simulink model "sim_tcyb_2024_att_ctrl"  (R2020a)
settings: Solver=ode4  StartTime=0.0  StopTime=30.0  FixedStep=0.01  RelTol=1e-3
values from neighbouring files (symbols this model uses):
  c1_diff_sigma_bar_w = diag([12; 12; 12])    [init_tcyb_2024_att_ctrl.m]
  c1_diff_ui = diag([25; 30; 20])    [init_tcyb_2024_att_ctrl.m]
  c2_diff_sigma_bar_w = diag([12; 12; 12])    [init_tcyb_2024_att_ctrl.m]
  c2_diff_ui = diag([50; 50; 10])    [init_tcyb_2024_att_ctrl.m]
  c3_diff_sigma_bar_w = diag([15; 15; 15])    [init_tcyb_2024_att_ctrl.m]
  c3_diff_ui = diag([15; 15; 10])    [init_tcyb_2024_att_ctrl.m]
  dw_aa_t = 0.2 * ones(3, 5) + ( 1.0 - 0.2 ) * rand(3, 5)    [init_tcyb_2024_att_ctrl.m]
  dw_ff_t = [ 0.4 * ones(1, 5) + ( 1.0 - 0.4 ) * rand(1, 5);                      0.4 * ones(1, 5) + ( 1.0 - 0.4 ) * rand(1, 5);                      0.2 * ones(1, 5) + ( 0.6 - 0.2 ) * rand(1, 5) ]    [init_tcyb_2024_att_ctrl.m]
  dw_phi_t = ( - pi / 2 ) * ones(3, 5) + ( pi / 2 - ( - pi / 2 ) ) * rand(3, 5)    [init_tcyb_2024_att_ctrl.m]
  dwci_init = zeros(3,NF)    [init_tcyb_2024_att_ctrl.m]
  h1w = diag([20.0; 20.0; 20.0])    [init_tcyb_2024_att_ctrl.m]
  h2w = diag([30.0; 35.0; 35.0])    [init_tcyb_2024_att_ctrl.m]
  h3w = diag([30.0; 25.0; 30.0])    [init_tcyb_2024_att_ctrl.m]
  Ji = zeros(3,3,NF)    [init_tcyb_2024_att_ctrl.m]
  ksg = diag([10.0, 10.0, 8.0])    [init_tcyb_2024_att_ctrl.m]
  kw = diag([10.0, 10.0, 8.0])    [init_tcyb_2024_att_ctrl.m]
  l1 = diag([5.0, 5.0, 4.0])    [init_tcyb_2024_att_ctrl.m]
  l2 = diag([5.0, 5.0, 4.0])    [init_tcyb_2024_att_ctrl.m]
  Lamd_diff_sigma_bar_w = 0.8    [init_tcyb_2024_att_ctrl.m]
  Lamd_diff_ui = 0.8    [init_tcyb_2024_att_ctrl.m]
  mu = diag([10.0, 10.0, 10.0, 8.0, 8.0, 8.0])    [init_tcyb_2024_att_ctrl.m]
  mu_d_w = 100    [init_tcyb_2024_att_ctrl.m]
  pos0 = zeros(3, 1)    [init_tcyb_2024_att_ctrl.m]
  PZ0 = P0(3)    [init_tcyb_2024_att_ctrl.m]
  PZ1 = 10    [init_tcyb_2024_att_ctrl.m]
  R0 = 4    [init_tcyb_2024_att_ctrl.m]
  R1 = 8    [init_tcyb_2024_att_ctrl.m]
  Rei_init = zeros(3,3,NF)    [init_tcyb_2024_att_ctrl.m]
  Ri_init = zeros(3,3,NF)    [init_tcyb_2024_att_ctrl.m]
  Rx2 = 10    [init_tcyb_2024_att_ctrl.m]
  Ry2 = 6    [init_tcyb_2024_att_ctrl.m]
  Rz2 = 4    [init_tcyb_2024_att_ctrl.m]
  sgei_init = zeros(3,NF)    [init_tcyb_2024_att_ctrl.m]
  sgi_init = zeros(3,NF)    [init_tcyb_2024_att_ctrl.m]
  T0 = 0    [init_tcyb_2024_att_ctrl.m]
  T1 = tseq1    (= 10)    [init_tcyb_2024_att_ctrl.m]
  T2 = tseq1 + tseq12 + tseq2    (= 30)    [init_tcyb_2024_att_ctrl.m]
  ui_init = zeros(3,NF)    [init_tcyb_2024_att_ctrl.m]
  V_Phi_Rei_init = zeros(3,NF)    [init_tcyb_2024_att_ctrl.m]
  vel0 = zeros(3, 1)    [init_tcyb_2024_att_ctrl.m]
  wci_init = zeros(3,NF)    [init_tcyb_2024_att_ctrl.m]
  wei_init = zeros(3,NF)    [init_tcyb_2024_att_ctrl.m]
  zeta_diff_sigma_bar_w = 0.3    [init_tcyb_2024_att_ctrl.m]
  zeta_diff_ui = 0.05    [init_tcyb_2024_att_ctrl.m]
undefined symbols (not defined in the file or in its folder): cal_frac_squ, p_alfaw1, p_alfaw2, q_alfaw1, q_alfaw2, wi_init
(part 3 of 5)

== matlab function sim_tcyb_2024_att_ctrl/combine Gamma_wi_vec ==
  data: Gamma_wi_1 input; Gamma_wi_2 input; Gamma_wi_3 input; Gamma_wi_4 input; Gamma_wi_5 input; Gamma_wi_vec output
function Gamma_wi_vec  = fcn(Gamma_wi_1, Gamma_wi_2, Gamma_wi_3, Gamma_wi_4, Gamma_wi_5)
%%%% 合并计算矩阵 Gamma_wi
Gamma_wi_vec = zeros(3,6,5);
Gamma_wi_vec(:,:,1) = Gamma_wi_1;
Gamma_wi_vec(:,:,2) = Gamma_wi_2;
Gamma_wi_vec(:,:,3) = Gamma_wi_3;
Gamma_wi_vec(:,:,4) = Gamma_wi_4;
Gamma_wi_vec(:,:,5) = Gamma_wi_5;

== matlab function sim_tcyb_2024_att_ctrl/cal Fi agent 1 ==
  data: wei_vec input; Fi_1 output; Rei_vec input; wci_vec input; dwci_vec input
function Fi_1 = fcn(wei_vec, Rei_vec, wci_vec, dwci_vec)
%%%% 计算补偿向量 Fi
iiuav = 1;
Fi_1 = cal_askew_mat( wei_vec(:,iiuav) ) * ( Rei_vec(:,:,iiuav)' ) * wci_vec(:,iiuav) ...
            - ( Rei_vec(:,:,iiuav)' ) * dwci_vec(:,iiuav);
end

== matlab function sim_tcyb_2024_att_ctrl/cal Fi agent 2 ==
  data: wei_vec input; Fi_2 output; Rei_vec input; wci_vec input; dwci_vec input
function Fi_2 = fcn(wei_vec, Rei_vec, wci_vec, dwci_vec)
%%%% 计算补偿向量 Fi
iiuav = 2;
Fi_2 = cal_askew_mat( wei_vec(:,iiuav) ) * ( Rei_vec(:,:,iiuav)' ) * wci_vec(:,iiuav) ...
            - ( Rei_vec(:,:,iiuav)' ) * dwci_vec(:,iiuav);
end

== matlab function sim_tcyb_2024_att_ctrl/combine wci dwci ==
  data: wci_node_1 input; wci_vec output; wci_node_2 input; wci_node_3 input; wci_node_4 input; wci_node_5 input; dwci_vec output; dwci_node_1 input; dwci_node_2 input; dwci_node_3 input; dwci_node_4 input; dwci_node_5 input
function [wci_vec, dwci_vec] = fcn(wci_node_1, wci_node_2, wci_node_3, wci_node_4, wci_node_5, ...
                                                                dwci_node_1, dwci_node_2, dwci_node_3, dwci_node_4, dwci_node_5)
%%%% 合并姿态角速率指令及其导数
wci_vec = [wci_node_1(:), wci_node_2(:), wci_node_3(:), wci_node_4(:), wci_node_5(:)];
dwci_vec = [dwci_node_1(:), dwci_node_2(:), dwci_node_3(:), dwci_node_4(:), dwci_node_5(:)];

== matlab function sim_tcyb_2024_att_ctrl/cal abs 11 ==
  data: x input; y output
function y = fcn(x)
y = abs(x(:));

== matlab function sim_tcyb_2024_att_ctrl/cal abs 12 ==
  data: x input; y output
function y = fcn(x)
y = abs(x(:));

== matlab function sim_tcyb_2024_att_ctrl/cal abs 13 ==
  data: x input; y output
function y = fcn(x)
y = abs(x(:));

== matlab function sim_tcyb_2024_att_ctrl/cal abs 14 ==
  data: x input; y output
function y = fcn(x)
y = abs(x(:));

== matlab function sim_tcyb_2024_att_ctrl/E_sgi agent 1 ==
  data: sgi_vec input; E_sgi_1 output
function E_sgi_1 = fcn(sgi_vec)
%%%% 更新四元数微分方程
iiuav = 1;
E_sgi_1 = (1/4) * ( ( 1 - (sgi_vec(:,iiuav)') * sgi_vec(:,iiuav) ) * eye(3) ...
                    + 2 * cal_askew_mat( sgi_vec(:,iiuav) ) + 2 * sgi_vec(:,iiuav) * ( sgi_vec(:,iiuav)' ) );
end

== matlab function sim_tcyb_2024_att_ctrl/cal abs 15 ==
  data: x input; y output
function y = fcn(x)
y = abs(x(:));

== matlab function sim_tcyb_2024_att_ctrl/cal abs 16 ==
  data: x input; y output
function y = fcn(x)
y = abs(x(:));

== matlab function sim_tcyb_2024_att_ctrl/cal abs 17 ==
  data: x input; y output
function y = fcn(x)
y = abs(x(:));

== matlab function sim_tcyb_2024_att_ctrl/cal abs 18 ==
  data: x input; y output
function y = fcn(x)
y = abs(x(:));

== matlab function sim_tcyb_2024_att_ctrl/combine tau ==
  data: tau_1 input; taui_vec output; tau_2 input; tau_3 input; tau_4 input; tau_5 input
function taui_vec = fcn(tau_1, tau_2, tau_3, tau_4, tau_5)
%%%% 合并辅助姿态角速率
taui_vec = [tau_1(:), tau_2(:), tau_3(:), tau_4(:), tau_5(:)];

== matlab function sim_tcyb_2024_att_ctrl/wi dynam agent 1 ==
  data: Ji input; dwi_1 output; wi_vec input; taui_vec input; dw_vec input
function dwi_1 = fcn(Ji, wi_vec, taui_vec, dw_vec)
%%%% 更新姿态角速率微分方程
iiuav = 1;
dwi_1 = inv(Ji(:,:,iiuav)) * ( -cal_askew_mat(wi_vec(:,iiuav)) * Ji(:,:,iiuav) * wi_vec(:,iiuav) ... 
                                                + taui_vec(:,iiuav) + dw_vec(:,iiuav) );

end

== matlab function sim_tcyb_2024_att_ctrl/cal abs 19 ==
  data: x input; y output
function y = fcn(x)
y = abs(x(:));

== matlab function sim_tcyb_2024_att_ctrl/cal abs 20 ==
  data: x input; y output
function y = fcn(x)
y = abs(x(:));

== matlab function sim_tcyb_2024_att_ctrl/cal d_sigma_w agent 1 ==
  data: h3w input; d_sigma_w_1 output; Ji input; wi_vec input; taui_vec input; sigma_w_bar_vec input
function d_sigma_w_1 = fcn(h3w, Ji, wi_vec, taui_vec, sigma_w_bar_vec)
%%%% 计算辅助姿态角速率导数
iiuav = 1;
d_sigma_w_1 = inv(Ji(:,:,iiuav)) * ( -cal_askew_mat(wi_vec(:,iiuav)) * Ji(:,:,iiuav) * wi_vec(:,iiuav) ...
                            + taui_vec(:,iiuav) + h3w * sigma_w_bar_vec(:,iiuav) );

== matlab function sim_tcyb_2024_att_ctrl/cal Ri agent 2 ==
  data: Ri_2 output; sgi_vec input
function Ri_2 = fcn(sgi_vec)
%%%% 由罗德里格常量sgi求解姿态旋转矩阵Ri
iiuav = 2;
Ri_2 = eye(3) + 4 * ( 1 - ( ( ( sgi_vec(:,iiuav)' ) * sgi_vec(:,iiuav) ) / ( ( 1 + ( sgi_vec(:,iiuav)' ) * sgi_vec(:,iiuav) ) ^ 2 ) ) ) * cal_askew_mat( sgi_vec(:,iiuav) ) ...
                            + ( 8 / ( ( 1 + ( sgi_vec(:,iiuav)' ) * sgi_vec(:,iiuav) ) ^ 2 ) ) * cal_askew_mat( sgi_vec(:,iiuav) ) * cal_askew_mat( sgi_vec(:,iiuav) );
Ri_2 = Ri_2';
end

== matlab function sim_tcyb_2024_att_ctrl/cal d_sigma_w agent 2 ==
  data: h3w input; d_sigma_w_2 output; Ji input; wi_vec input; taui_vec input; sigma_w_bar_vec input
function d_sigma_w_2 = fcn(h3w, Ji, wi_vec, taui_vec, sigma_w_bar_vec)
%%%% 计算辅助姿态角速率导数
iiuav = 2;
d_sigma_w_2 = inv(Ji(:,:,iiuav)) * ( -cal_askew_mat(wi_vec(:,iiuav)) * Ji(:,:,iiuav) * wi_vec(:,iiuav) ...
                            + taui_vec(:,iiuav) + h3w * sigma_w_bar_vec(:,iiuav) );

== matlab function sim_tcyb_2024_att_ctrl/cal d_sigma_w agent 3 ==
  data: h3w input; d_sigma_w_3 output; Ji input; wi_vec input; taui_vec input; sigma_w_bar_vec input
function d_sigma_w_3 = fcn(h3w, Ji, wi_vec, taui_vec, sigma_w_bar_vec)
%%%% 计算辅助姿态角速率导数
iiuav = 3;
d_sigma_w_3 = inv(Ji(:,:,iiuav)) * ( -cal_askew_mat(wi_vec(:,iiuav)) * Ji(:,:,iiuav) * wi_vec(:,iiuav) ...
                            + taui_vec(:,iiuav) + h3w * sigma_w_bar_vec(:,iiuav) );

== matlab function sim_tcyb_2024_att_ctrl/cal d_sigma_w agent 4 ==
  data: h3w input; d_sigma_w_4 output; Ji input; wi_vec input; taui_vec input; sigma_w_bar_vec input
function d_sigma_w_4 = fcn(h3w, Ji, wi_vec, taui_vec, sigma_w_bar_vec)
%%%% 计算辅助姿态角速率导数
iiuav = 4;
d_sigma_w_4 = inv(Ji(:,:,iiuav)) * ( -cal_askew_mat(wi_vec(:,iiuav)) * Ji(:,:,iiuav) * wi_vec(:,iiuav) ...
                            + taui_vec(:,iiuav) + h3w * sigma_w_bar_vec(:,iiuav) );

== matlab function sim_tcyb_2024_att_ctrl/wi dynam agent 2 ==
  data: Ji input; dwi_2 output; wi_vec input; taui_vec input; dw_vec input
function dwi_2 = fcn(Ji, wi_vec, taui_vec, dw_vec)
%%%% 更新姿态角速率微分方程
iiuav = 2;
dwi_2 = inv(Ji(:,:,iiuav)) * ( -cal_askew_mat(wi_vec(:,iiuav)) * Ji(:,:,iiuav) * wi_vec(:,iiuav) ... 
                                                + taui_vec(:,iiuav) + dw_vec(:,iiuav) );

end

== matlab function sim_tcyb_2024_att_ctrl/wi dynam agent 3 ==
  data: Ji input; dwi_3 output; wi_vec input; taui_vec input; dw_vec input
function dwi_3 = fcn(Ji, wi_vec, taui_vec, dw_vec)
%%%% 更新姿态角速率微分方程
iiuav = 3;
dwi_3 = inv(Ji(:,:,iiuav)) * ( -cal_askew_mat(wi_vec(:,iiuav)) * Ji(:,:,iiuav) * wi_vec(:,iiuav) ...
                                                + taui_vec(:,iiuav) + dw_vec(:,iiuav) );

end

== matlab function sim_tcyb_2024_att_ctrl/wi dynam agent 4 ==
  data: Ji input; dwi_4 output; wi_vec input; taui_vec input; dw_vec input
function dwi_4 = fcn(Ji, wi_vec, taui_vec, dw_vec)
%%%% 更新姿态角速率微分方程
iiuav = 4;
dwi_4 = inv(Ji(:,:,iiuav)) * ( -cal_askew_mat(wi_vec(:,iiuav)) * Ji(:,:,iiuav) * wi_vec(:,iiuav) ...
                                                + taui_vec(:,iiuav) + dw_vec(:,iiuav) );

end

== matlab function sim_tcyb_2024_att_ctrl/E_sgi agent 2 ==
  data: sgi_vec input; E_sgi_2 output
function E_sgi_2 = fcn(sgi_vec)
%%%% 更新四元数微分方程
iiuav = 2;
E_sgi_2 = (1/4) * ( ( 1 - (sgi_vec(:,iiuav)') * sgi_vec(:,iiuav) ) * eye(3) ...
                    + 2 * cal_askew_mat( sgi_vec(:,iiuav) ) + 2 * sgi_vec(:,iiuav) * ( sgi_vec(:,iiuav)' ) );
end

== matlab function sim_tcyb_2024_att_ctrl/wi dynam agent 5 ==
  data: Ji input; dwi_5 output; wi_vec input; taui_vec input; dw_vec input
function dwi_5 = fcn(Ji, wi_vec, taui_vec, dw_vec)
%%%% 更新姿态角速率微分方程
iiuav = 5;
dwi_5 = inv(Ji(:,:,iiuav)) * ( -cal_askew_mat(wi_vec(:,iiuav)) * Ji(:,:,iiuav) * wi_vec(:,iiuav) ...
                                                + taui_vec(:,iiuav) + dw_vec(:,iiuav) );

end

== matlab function sim_tcyb_2024_att_ctrl/combine dwi ==
  data: wi_1 input; wi_vec output; wi_2 input; wi_3 input; wi_4 input; wi_5 input
function wi_vec = fcn(wi_1, wi_2, wi_3, wi_4, wi_5)
%%%% 合并姿态角速率
wi_vec = [wi_1(:), wi_2(:), wi_3(:), wi_4(:), wi_5(:)];

== matlab function sim_tcyb_2024_att_ctrl/sgi dynam agent 1 ==
  data: E_sgi_vec input; dsgi_1 output; wi_vec input
function dsgi_1 = fcn(E_sgi_vec, wi_vec)
%%%% 更新四元数微分方程
iiuav = 1;
dsgi_1 = E_sgi_vec(:,:,iiuav) * wi_vec(:,iiuav);
end

== matlab function sim_tcyb_2024_att_ctrl/cal Fi agent 3 ==
  data: wei_vec input; Fi_3 output; Rei_vec input; wci_vec input; dwci_vec input
function Fi_3 = fcn(wei_vec, Rei_vec, wci_vec, dwci_vec)
%%%% 计算补偿向量 Fi
iiuav = 3;
Fi_3 = cal_askew_mat( wei_vec(:,iiuav) ) * ( Rei_vec(:,:,iiuav)' ) * wci_vec(:,iiuav) ...
            - ( Rei_vec(:,:,iiuav)' ) * dwci_vec(:,iiuav);
end

== matlab function sim_tcyb_2024_att_ctrl/cal d_sigma_w agent 5 ==
  data: h3w input; d_sigma_w_5 output; Ji input; wi_vec input; taui_vec input; sigma_w_bar_vec input
function d_sigma_w_5 = fcn(h3w, Ji, wi_vec, taui_vec, sigma_w_bar_vec)
%%%% 计算辅助姿态角速率导数
iiuav = 5;
d_sigma_w_5 = inv(Ji(:,:,iiuav)) * ( -cal_askew_mat(wi_vec(:,iiuav)) * Ji(:,:,iiuav) * wi_vec(:,iiuav) ...
                            + taui_vec(:,iiuav) + h3w * sigma_w_bar_vec(:,iiuav) );

== matlab function sim_tcyb_2024_att_ctrl/cal differentiator d_sigma_bar_w_hat agent 1/cal differentiator ==
  data: c1 input; d_sigma_bar_v_hat output; d_dsigma_bar_v_hat output; d_d2sigma_bar_v_hat output; c2 input; c3 input; chi_t input; sigma_bar_v_sig_1 input; sigma_bar_v_sig_2 input; sigma_bar_v_sig_3 input; sigma_bar_v_sig_4 input; sigma_bar_v_sig_5 input; sigma_bar_v_sig_6 input; d_sigma_bar_v_hat input; d2_sigma_bar_v_hat input
function [d_sigma_bar_v_hat, d_dsigma_bar_v_hat, d_d2sigma_bar_v_hat] = fcn(c1, c2, c3, chi_t, sigma_bar_v_sig_1, sigma_bar_v_sig_2, sigma_bar_v_sig_3, ...
                                                                                                                                                sigma_bar_v_sig_4, sigma_bar_v_sig_5, sigma_bar_v_sig_6, d_sigma_bar_v_hat, d2_sigma_bar_v_hat)
d_d2sigma_bar_v_hat = -chi_t .* c1 * sigma_bar_v_sig_1(:) - (1 - chi_t) .* c1 * sigma_bar_v_sig_2(:);
d_dsigma_bar_v_hat = -chi_t .* c2 * sigma_bar_v_sig_3(:) - (1 - chi_t) .* c2 * sigma_bar_v_sig_4(:) + d2_sigma_bar_v_hat(:);
d_sigma_bar_v_hat = -chi_t .* c3 * sigma_bar_v_sig_5(:) - (1 - chi_t) .* c3 * sigma_bar_v_sig_6(:) + d_sigma_bar_v_hat(:);

== matlab function sim_tcyb_2024_att_ctrl/sgi dynam agent 2 ==
  data: E_sgi_vec input; dsgi_2 output; wi_vec input
function dsgi_2 = fcn(E_sgi_vec, wi_vec)
%%%% 更新四元数微分方程
iiuav = 2;
dsgi_2 = E_sgi_vec(:,:,iiuav) * wi_vec(:,iiuav);
end

== matlab function sim_tcyb_2024_att_ctrl/cal differentiator d_sigma_bar_w_hat agent 1/cal sig ==
  data: x input; z output; y input
function z = fcn(x, y)
z = x(:) .* sign(y(:));

== matlab function sim_tcyb_2024_att_ctrl/cal differentiator d_sigma_bar_w_hat agent 1/cal sig1 ==
  data: x input; z output; y input
function z = fcn(x, y)
z = x(:) .* sign(y(:));

== matlab function sim_tcyb_2024_att_ctrl/cal differentiator d_sigma_bar_w_hat agent 1/cal sig2 ==
  data: x input; z output; y input
function z = fcn(x, y)
z = x(:) .* sign(y(:));

== matlab function sim_tcyb_2024_att_ctrl/cal differentiator d_sigma_bar_w_hat agent 1/cal sig3 ==
  data: x input; z output; y input
function z = fcn(x, y)
z = x(:) .* sign(y(:));

== matlab function sim_tcyb_2024_att_ctrl/cal differentiator d_sigma_bar_w_hat agent 1/cal sig4 ==
  data: x input; z output; y input
function z = fcn(x, y)
z = x(:) .* sign(y(:));

== matlab function sim_tcyb_2024_att_ctrl/cal differentiator d_sigma_bar_w_hat agent 1/cal sig5 ==
  data: x input; z output; y input
function z = fcn(x, y)
z = x(:) .* sign(y(:));

== matlab function sim_tcyb_2024_att_ctrl/cal differentiator d_sigma_bar_w_hat agent 1/choose sigma_bar_w ==
  data: x input; y output
function y = fcn(x)
iiuav = 1;
y = x(:,iiuav);

== matlab function sim_tcyb_2024_att_ctrl/cal differentiator d_sigma_bar_w_hat agent 1/trans to column20 ==
  data: x input; y output
function y = fcn(x)
y = x(:);

== matlab function sim_tcyb_2024_att_ctrl/cal differentiator d_sigma_bar_w_hat agent 1/trans to column21 ==
  data: x input; y output
function y = fcn(x)
y = x(:);

== matlab function sim_tcyb_2024_att_ctrl/cal differentiator d_sigma_bar_w_hat agent 1/trans to column22 ==
  data: x input; y output
function y = fcn(x)
y = x(:);

== matlab function sim_tcyb_2024_att_ctrl/cal differentiator d_sigma_bar_w_hat agent 1/trans to column23 ==
  data: x input; y output
function y = fcn(x)
y = x(:);

== matlab function sim_tcyb_2024_att_ctrl/depart wc5 ==
  data: y output; x input
function y = fcn(x)
y = x(:,5);

end

== matlab function sim_tcyb_2024_att_ctrl/cal differentiator d_sigma_bar_w_hat agent 1/trans to column24 ==
  data: x input; y output
function y = fcn(x)
y = x(:);

== matlab function sim_tcyb_2024_att_ctrl/cal differentiator d_sigma_bar_w_hat agent 1/trans to column25 ==
  data: x input; y output
function y = fcn(x)
y = x(:);

== matlab function sim_tcyb_2024_att_ctrl/cal differentiator d_sigma_bar_w_hat agent 2/cal differentiator ==
  data: c1 input; d_sigma_bar_v_hat output; d_dsigma_bar_v_hat output; d_d2sigma_bar_v_hat output; c2 input; c3 input; chi_t input; sigma_bar_v_sig_1 input; sigma_bar_v_sig_2 input; sigma_bar_v_sig_3 input; sigma_bar_v_sig_4 input; sigma_bar_v_sig_5 input; sigma_bar_v_sig_6 input; d_sigma_bar_v_hat input; d2_sigma_bar_v_hat input
function [d_sigma_bar_v_hat, d_dsigma_bar_v_hat, d_d2sigma_bar_v_hat] = fcn(c1, c2, c3, chi_t, sigma_bar_v_sig_1, sigma_bar_v_sig_2, sigma_bar_v_sig_3, ...
                                                                                                                                                sigma_bar_v_sig_4, sigma_bar_v_sig_5, sigma_bar_v_sig_6, d_sigma_bar_v_hat, d2_sigma_bar_v_hat)
d_d2sigma_bar_v_hat = -chi_t .* c1 * sigma_bar_v_sig_1(:) - (1 - chi_t) .* c1 * sigma_bar_v_sig_2(:);
d_dsigma_bar_v_hat = -chi_t .* c2 * sigma_bar_v_sig_3(:) - (1 - chi_t) .* c2 * sigma_bar_v_sig_4(:) + d2_sigma_bar_v_hat(:);
d_sigma_bar_v_hat = -chi_t .* c3 * sigma_bar_v_sig_5(:) - (1 - chi_t) .* c3 * sigma_bar_v_sig_6(:) + d_sigma_bar_v_hat(:);

== matlab function sim_tcyb_2024_att_ctrl/cal differentiator d_sigma_bar_w_hat agent 2/cal sig ==
  data: x input; z output; y input
function z = fcn(x, y)
z = x(:) .* sign(y(:));

== matlab function sim_tcyb_2024_att_ctrl/cal differentiator d_sigma_bar_w_hat agent 2/cal sig1 ==
  data: x input; z output; y input
function z = fcn(x, y)
z = x(:) .* sign(y(:));

== matlab function sim_tcyb_2024_att_ctrl/cal differentiator d_sigma_bar_w_hat agent 2/cal sig2 ==
  data: x input; z output; y input
function z = fcn(x, y)
z = x(:) .* sign(y(:));

== matlab function sim_tcyb_2024_att_ctrl/cal differentiator d_sigma_bar_w_hat agent 2/cal sig3 ==
  data: x input; z output; y input
function z = fcn(x, y)
z = x(:) .* sign(y(:));

== matlab function sim_tcyb_2024_att_ctrl/depart wc1 ==
  data: y output; x input
function y = fcn(x)
y = x(:,1);

end

== matlab function sim_tcyb_2024_att_ctrl/cal differentiator d_sigma_bar_w_hat agent 2/cal sig4 ==
  data: x input; z output; y input
function z = fcn(x, y)
z = x(:) .* sign(y(:));

== matlab function sim_tcyb_2024_att_ctrl/cal differentiator d_sigma_bar_w_hat agent 2/cal sig5 ==
  data: x input; z output; y input
function z = fcn(x, y)
z = x(:) .* sign(y(:));

== matlab function sim_tcyb_2024_att_ctrl/cal differentiator d_sigma_bar_w_hat agent 2/choose sigma_bar_w ==
  data: x input; y output
function y = fcn(x)
iiuav = 2;
y = x(:,iiuav);

== matlab function sim_tcyb_2024_att_ctrl/cal differentiator d_sigma_bar_w_hat agent 2/trans to column20 ==
  data: x input; y output
function y = fcn(x)
y = x(:);

== matlab function sim_tcyb_2024_att_ctrl/cal differentiator d_sigma_bar_w_hat agent 2/trans to column21 ==
  data: x input; y output
function y = fcn(x)
y = x(:);

== matlab function sim_tcyb_2024_att_ctrl/cal differentiator d_sigma_bar_w_hat agent 2/trans to column22 ==
  data: x input; y output
function y = fcn(x)
y = x(:);

== matlab function sim_tcyb_2024_att_ctrl/cal differentiator d_sigma_bar_w_hat agent 2/trans to column23 ==
  data: x input; y output
function y = fcn(x)
y = x(:);

== matlab function sim_tcyb_2024_att_ctrl/cal taui agent 1 ==
  data: kw input; ksg input; tau_1 output; wi_vec input; wei_vec input; zetai_vec input; sgei_vec input; dw_hat_vec input; thetai_hat_vec input; Gamma_wi_vec input; Gamma_Fi_min_dzetai_vec input
function tau_1 = fcn(kw, ksg, wi_vec, wei_vec, zetai_vec, sgei_vec, dw_hat_vec, ...
                                        thetai_hat_vec, Gamma_wi_vec, Gamma_Fi_min_dzetai_vec)
%%%% 计算用于姿态控制的驱动力矩控制输入
iiuav = 1;
tau_1 = -kw * ( wei_vec(:,iiuav) - zetai_vec(:,iiuav) ) - ksg * sgei_vec(:,iiuav) - dw_hat_vec(:,iiuav) ...
                - ( Gamma_Fi_min_dzetai_vec(:,:,iiuav) - cal_askew_mat( wi_vec(:,iiuav) ) * Gamma_wi_vec(:,:,iiuav) ) * thetai_hat_vec(:,iiuav);
end

== matlab function sim_tcyb_2024_att_ctrl/cal Fi agent 4 ==
  data: wei_vec input; Fi_4 output; Rei_vec input; wci_vec input; dwci_vec input
function Fi_4 = fcn(wei_vec, Rei_vec, wci_vec, dwci_vec)
%%%% 计算补偿向量 Fi
iiuav = 4;
Fi_4 = cal_askew_mat( wei_vec(:,iiuav) ) * ( Rei_vec(:,:,iiuav)' ) * wci_vec(:,iiuav) ...
            - ( Rei_vec(:,:,iiuav)' ) * dwci_vec(:,iiuav);
end

== matlab function sim_tcyb_2024_att_ctrl/depart wc2 ==
  data: y output; x input
function y = fcn(x)
y = x(:,2);

end

== matlab function sim_tcyb_2024_att_ctrl/cal Fi agent 5 ==
  data: wei_vec input; Fi_5 output; Rei_vec input; wci_vec input; dwci_vec input
function Fi_5 = fcn(wei_vec, Rei_vec, wci_vec, dwci_vec)
%%%% 计算补偿向量 Fi
iiuav = 5;
Fi_5 = cal_askew_mat( wei_vec(:,iiuav) ) * ( Rei_vec(:,:,iiuav)' ) * wci_vec(:,iiuav) ...
            - ( Rei_vec(:,:,iiuav)' ) * dwci_vec(:,iiuav);
end

== matlab function sim_tcyb_2024_att_ctrl/combine Fi_vec ==
  data: Fi_1 input; Fi_2 input; Fi_3 input; Fi_4 input; Fi_5 input; Fi_vec output
function Fi_vec  = fcn(Fi_1, Fi_2, Fi_3, Fi_4, Fi_5)
%%%% 合并计算矩阵 Fi
Fi_vec = zeros(3,5);
Fi_vec(:,1) = Fi_1(:);
Fi_vec(:,2) = Fi_2(:);
Fi_vec(:,3) = Fi_3(:);
Fi_vec(:,4) = Fi_4(:);
Fi_vec(:,5) = Fi_5(:);

== matlab function sim_tcyb_2024_att_ctrl/combine sgi Ri ==
  data: sgi_1 input; sgi_vec output; sgi_2 input; sgi_3 input; sgi_4 input; sgi_5 input; Ri_1 input; Ri_2 input; Ri_3 input; Ri_4 input; Ri_5 input; Ri_vec output
function [sgi_vec, Ri_vec] = fcn(sgi_1, sgi_2, sgi_3, sgi_4, sgi_5, ...
                                                            Ri_1, Ri_2, Ri_3, Ri_4, Ri_5)
%%%% 合并四元数和姿态旋转矩阵
sgi_vec = zeros(3,5);
sgi_vec(:,1) = sgi_1(:);
sgi_vec(:,2) = sgi_2(:);
sgi_vec(:,3) = sgi_3(:);
sgi_vec(:,4) = sgi_4(:);
sgi_vec(:,5) = sgi_5(:);

Ri_vec = zeros(3,3,5);
Ri_vec(:,:,1) = Ri_1;
Ri_vec(:,:,2) = Ri_2;
Ri_vec(:,:,3) = Ri_3;
Ri_vec(:,:,4) = Ri_4;
Ri_vec(:,:,5) = Ri_5;

== matlab function sim_tcyb_2024_att_ctrl/cal differentiator d_sigma_bar_w_hat agent 2/trans to column24 ==
  data: x input; y output
function y = fcn(x)
y = x(:);

== matlab function sim_tcyb_2024_att_ctrl/cal differentiator d_sigma_bar_w_hat agent 2/trans to column25 ==
  data: x input; y output
function y = fcn(x)
y = x(:);

== matlab function sim_tcyb_2024_att_ctrl/cal differentiator d_sigma_bar_w_hat agent 3/cal differentiator ==
  data: c1 input; d_sigma_bar_v_hat output; d_dsigma_bar_v_hat output; d_d2sigma_bar_v_hat output; c2 input; c3 input; chi_t input; sigma_bar_v_sig_1 input; sigma_bar_v_sig_2 input; sigma_bar_v_sig_3 input; sigma_bar_v_sig_4 input; sigma_bar_v_sig_5 input; sigma_bar_v_sig_6 input; d_sigma_bar_v_hat input; d2_sigma_bar_v_hat input
function [d_sigma_bar_v_hat, d_dsigma_bar_v_hat, d_d2sigma_bar_v_hat] = fcn(c1, c2, c3, chi_t, sigma_bar_v_sig_1, sigma_bar_v_sig_2, sigma_bar_v_sig_3, ...
                                                                                                                                                sigma_bar_v_sig_4, sigma_bar_v_sig_5, sigma_bar_v_sig_6, d_sigma_bar_v_hat, d2_sigma_bar_v_hat)
d_d2sigma_bar_v_hat = -chi_t .* c1 * sigma_bar_v_sig_1(:) - (1 - chi_t) .* c1 * sigma_bar_v_sig_2(:);
d_dsigma_bar_v_hat = -chi_t .* c2 * sigma_bar_v_sig_3(:) - (1 - chi_t) .* c2 * sigma_bar_v_sig_4(:) + d2_sigma_bar_v_hat(:);
d_sigma_bar_v_hat = -chi_t .* c3 * sigma_bar_v_sig_5(:) - (1 - chi_t) .* c3 * sigma_bar_v_sig_6(:) + d_sigma_bar_v_hat(:);

== matlab function sim_tcyb_2024_att_ctrl/depart wc3 ==
  data: y output; x input
function y = fcn(x)
y = x(:,3);

end

== matlab function sim_tcyb_2024_att_ctrl/cal differentiator d_sigma_bar_w_hat agent 3/cal sig ==
  data: x input; z output; y input
function z = fcn(x, y)
z = x(:) .* sign(y(:));

== matlab function sim_tcyb_2024_att_ctrl/cal differentiator d_sigma_bar_w_hat agent 3/cal sig1 ==
  data: x input; z output; y input
function z = fcn(x, y)
z = x(:) .* sign(y(:));

== matlab function sim_tcyb_2024_att_ctrl/cal Gamma_Fi agent 2 ==
  data: Fi_vec input; Gamma_Fi_2 output
function Gamma_Fi_2 = fcn(Fi_vec)
%%%% 计算矩阵 Gamma_Fi
iiuav = 2;
Gamma_Fi_2 = [Fi_vec(1,iiuav), 0, 0, 0, Fi_vec(3,iiuav), Fi_vec(2,iiuav); ...
                                0, Fi_vec(2,iiuav), 0, Fi_vec(3,iiuav), 0, Fi_vec(1,iiuav); ...
                                0, 0, Fi_vec(3,iiuav), Fi_vec(2,iiuav), Fi_vec(1,iiuav), 0];
end

== matlab function sim_tcyb_2024_att_ctrl/cal differentiator d_sigma_bar_w_hat agent 3/cal sig2 ==
  data: x input; z output; y input
function z = fcn(x, y)
z = x(:) .* sign(y(:));

== matlab function sim_tcyb_2024_att_ctrl/cal Gamma_Fi agent 1 ==
  data: Fi_vec input; Gamma_Fi_1 output
function Gamma_Fi_1 = fcn(Fi_vec)
%%%% 计算矩阵 Gamma_Fi
iiuav = 1;
Gamma_Fi_1 = [Fi_vec(1,iiuav), 0, 0, 0, Fi_vec(3,iiuav), Fi_vec(2,iiuav); ...
                                0, Fi_vec(2,iiuav), 0, Fi_vec(3,iiuav), 0, Fi_vec(1,iiuav); ...
                                0, 0, Fi_vec(3,iiuav), Fi_vec(2,iiuav), Fi_vec(1,iiuav), 0];
end

== matlab function sim_tcyb_2024_att_ctrl/cal Gamma_Fi agent 3 ==
  data: Fi_vec input; Gamma_Fi_3 output
function Gamma_Fi_3 = fcn(Fi_vec)
%%%% 计算矩阵 Gamma_Fi
iiuav = 3;
Gamma_Fi_3 = [Fi_vec(1,iiuav), 0, 0, 0, Fi_vec(3,iiuav), Fi_vec(2,iiuav); ...
                                0, Fi_vec(2,iiuav), 0, Fi_vec(3,iiuav), 0, Fi_vec(1,iiuav); ...
                                0, 0, Fi_vec(3,iiuav), Fi_vec(2,iiuav), Fi_vec(1,iiuav), 0];
end

== matlab function sim_tcyb_2024_att_ctrl/cal Gamma_Fi agent 4 ==
  data: Fi_vec input; Gamma_Fi_4 output
function Gamma_Fi_4 = fcn(Fi_vec)
%%%% 计算矩阵 Gamma_Fi
iiuav = 4;
Gamma_Fi_4 = [Fi_vec(1,iiuav), 0, 0, 0, Fi_vec(3,iiuav), Fi_vec(2,iiuav); ...
                                0, Fi_vec(2,iiuav), 0, Fi_vec(3,iiuav), 0, Fi_vec(1,iiuav); ...
                                0, 0, Fi_vec(3,iiuav), Fi_vec(2,iiuav), Fi_vec(1,iiuav), 0];
end

== matlab function sim_tcyb_2024_att_ctrl/cal Gamma_Fi agent 5 ==
  data: Fi_vec input; Gamma_Fi_5 output
function Gamma_Fi_5 = fcn(Fi_vec)
%%%% 计算矩阵 Gamma_Fi
iiuav = 5;
Gamma_Fi_5 = [Fi_vec(1,iiuav), 0, 0, 0, Fi_vec(3,iiuav), Fi_vec(2,iiuav); ...
                                0, Fi_vec(2,iiuav), 0, Fi_vec(3,iiuav), 0, Fi_vec(1,iiuav); ...
                                0, 0, Fi_vec(3,iiuav), Fi_vec(2,iiuav), Fi_vec(1,iiuav), 0];
end

== matlab function sim_tcyb_2024_att_ctrl/combine Gamma_Fi_vec ==
  data: Gamma_Fi_1 input; Gamma_Fi_2 input; Gamma_Fi_3 input; Gamma_Fi_4 input; Gamma_Fi_5 input; Gamma_Fi_vec output
function Gamma_Fi_vec  = fcn(Gamma_Fi_1, Gamma_Fi_2, Gamma_Fi_3, Gamma_Fi_4, Gamma_Fi_5)
%%%% 合并计算矩阵 Gamma_Fi
Gamma_Fi_vec = zeros(3,6,5);
Gamma_Fi_vec(:,:,1) = Gamma_Fi_1;
Gamma_Fi_vec(:,:,2) = Gamma_Fi_2;
Gamma_Fi_vec(:,:,3) = Gamma_Fi_3;
Gamma_Fi_vec(:,:,4) = Gamma_Fi_4;
Gamma_Fi_vec(:,:,5) = Gamma_Fi_5;

== matlab function sim_tcyb_2024_att_ctrl/depart wc4 ==
  data: y output; x input
function y = fcn(x)
y = x(:,4);

end

== matlab function sim_tcyb_2024_att_ctrl/cal zetai agent 1 ==
  data: l1 input; d_zetai_1 output; l2 input; ksg input; zetai_vec input; sgei_vec input
function d_zetai_1 = fcn(l1, l2, ksg, zetai_vec, sgei_vec)
%%%% 计算自适应律 d_zetai
iiuav = 1;
d_zetai_1 = -l1 * zetai_vec(:,iiuav) - l2 * ksg * sgei_vec(:,iiuav);
end

== matlab function sim_tcyb_2024_att_ctrl/cal zetai agent 2 ==
  data: l1 input; d_zetai_2 output; l2 input; ksg input; zetai_vec input; sgei_vec input
function d_zetai_2 = fcn(l1, l2, ksg, zetai_vec, sgei_vec)
%%%% 计算自适应律 d_zetai
iiuav = 2;
d_zetai_2 = -l1 * zetai_vec(:,iiuav) - l2 * ksg * sgei_vec(:,iiuav);
end

== matlab function sim_tcyb_2024_att_ctrl/cal zetai agent 3 ==
  data: l1 input; d_zetai_3 output; l2 input; ksg input; zetai_vec input; sgei_vec input
function d_zetai_3 = fcn(l1, l2, ksg, zetai_vec, sgei_vec)
%%%% 计算自适应律 d_zetai
iiuav = 3;
d_zetai_3 = -l1 * zetai_vec(:,iiuav) - l2 * ksg * sgei_vec(:,iiuav);
end

== matlab function sim_tcyb_2024_att_ctrl/cal zetai agent 4 ==
  data: l1 input; d_zetai_4 output; l2 input; ksg input; zetai_vec input; sgei_vec input
function d_zetai_4 = fcn(l1, l2, ksg, zetai_vec, sgei_vec)
%%%% 计算自适应律 d_zetai
iiuav = 4;
d_zetai_4 = -l1 * zetai_vec(:,iiuav) - l2 * ksg * sgei_vec(:,iiuav);
end

== matlab function sim_tcyb_2024_att_ctrl/cal zetai agent 5 ==
  data: l1 input; d_zetai_5 output; l2 input; ksg input; zetai_vec input; sgei_vec input
function d_zetai_5 = fcn(l1, l2, ksg, zetai_vec, sgei_vec)
%%%% 计算自适应律 d_zetai
iiuav = 5;
d_zetai_5 = -l1 * zetai_vec(:,iiuav) - l2 * ksg * sgei_vec(:,iiuav);
end

== matlab function sim_tcyb_2024_att_ctrl/combine zetai_vec ==
  data: zetai_1 input; zetai_2 input; zetai_3 input; zetai_4 input; zetai_5 input; zetai_vec output
function zetai_vec  = fcn(zetai_1, zetai_2, zetai_3, zetai_4, zetai_5)
%%%% 合并自适应变量 zetai
zetai_vec = zeros(3,5);
zetai_vec(:,1) = zetai_1(:);
zetai_vec(:,2) = zetai_2(:);
zetai_vec(:,3) = zetai_3(:);
zetai_vec(:,4) = zetai_4(:);
zetai_vec(:,5) = zetai_5(:);

== matlab function sim_tcyb_2024_att_ctrl/E_sgei agent 1 ==
  data: sgei_vec input; E_sgei_1 output
function E_sgei_1 = fcn(sgei_vec)
%%%% 更新四元数微分方程
iiuav = 1;
E_sgei_1 = (1/4) * ( ( 1 - (sgei_vec(:,iiuav)') * sgei_vec(:,iiuav) ) * eye(3) ...
                    + 2 * cal_askew_mat( sgei_vec(:,iiuav) ) + 2 * sgei_vec(:,iiuav) * ( sgei_vec(:,iiuav)' ) );
end

== matlab function sim_tcyb_2024_att_ctrl/combine d_zetai_vec ==
  data: d_zetai_1 input; d_zetai_2 input; d_zetai_3 input; d_zetai_4 input; d_zetai_5 input; d_zetai_vec output
function d_zetai_vec  = fcn(d_zetai_1, d_zetai_2, d_zetai_3, d_zetai_4, d_zetai_5)
%%%% 合并自适应变量导数 d_zetai
d_zetai_vec = zeros(3,5);
d_zetai_vec(:,1) = d_zetai_1(:);
d_zetai_vec(:,2) = d_zetai_2(:);
d_zetai_vec(:,3) = d_zetai_3(:);
d_zetai_vec(:,4) = d_zetai_4(:);
d_zetai_vec(:,5) = d_zetai_5(:);

== matlab function sim_tcyb_2024_att_ctrl/cal Gamma_Fi_min_dzetai agent 1 ==
  data: Gamma_Fi_vec input; Gamma_Fi_min_dzetai_1 output; d_zetai_vec input
function Gamma_Fi_min_dzetai_1 = fcn(Gamma_Fi_vec, d_zetai_vec)
%%%% 计算矩阵 Gamma_Fi_min_dzetai
iiuav = 1;
Gamma_Fi_min_dzetai_1 = zeros(3,6);
Gamma_Fi_min_dzetai_1(1,1) = Gamma_Fi_vec(1,1) - d_zetai_vec(1,iiuav);
Gamma_Fi_min_dzetai_1(2,2) = Gamma_Fi_vec(2,2) - d_zetai_vec(2,iiuav);
Gamma_Fi_min_dzetai_1(3,3) = Gamma_Fi_vec(3,3) - d_zetai_vec(3,iiuav);
Gamma_Fi_min_dzetai_1(2,4) = Gamma_Fi_vec(2,4) - d_zetai_vec(3,iiuav);
Gamma_Fi_min_dzetai_1(3,4) = Gamma_Fi_vec(3,4) - d_zetai_vec(2,iiuav);
Gamma_Fi_min_dzetai_1(1,5) = Gamma_Fi_vec(1,5) - d_zetai_vec(3,iiuav);
Gamma_Fi_min_dzetai_1(3,5) = Gamma_Fi_vec(3,5) - d_zetai_vec(1,iiuav);
Gamma_Fi_min_dzetai_1(1,6) = Gamma_Fi_vec(1,6) - d_zetai_vec(2,iiuav);
Gamma_Fi_min_dzetai_1(2,6) = Gamma_Fi_vec(2,6) - d_zetai_vec(1,iiuav);
end

== matlab function sim_tcyb_2024_att_ctrl/cal Gamma_Fi_min_dzetai agent 2 ==
  data: Gamma_Fi_vec input; Gamma_Fi_min_dzetai_2 output; d_zetai_vec input
function Gamma_Fi_min_dzetai_2 = fcn(Gamma_Fi_vec, d_zetai_vec)
%%%% 计算矩阵 Gamma_Fi_min_dzetai
iiuav = 2;
Gamma_Fi_min_dzetai_2 = zeros(3,6);
Gamma_Fi_min_dzetai_2(1,1) = Gamma_Fi_vec(1,1) - d_zetai_vec(1,iiuav);
Gamma_Fi_min_dzetai_2(2,2) = Gamma_Fi_vec(2,2) - d_zetai_vec(2,iiuav);
Gamma_Fi_min_dzetai_2(3,3) = Gamma_Fi_vec(3,3) - d_zetai_vec(3,iiuav);
Gamma_Fi_min_dzetai_2(2,4) = Gamma_Fi_vec(2,4) - d_zetai_vec(3,iiuav);
Gamma_Fi_min_dzetai_2(3,4) = Gamma_Fi_vec(3,4) - d_zetai_vec(2,iiuav);
Gamma_Fi_min_dzetai_2(1,5) = Gamma_Fi_vec(1,5) - d_zetai_vec(3,iiuav);
Gamma_Fi_min_dzetai_2(3,5) = Gamma_Fi_vec(3,5) - d_zetai_vec(1,iiuav);
Gamma_Fi_min_dzetai_2(1,6) = Gamma_Fi_vec(1,6) - d_zetai_vec(2,iiuav);
Gamma_Fi_min_dzetai_2(2,6) = Gamma_Fi_vec(2,6) - d_zetai_vec(1,iiuav);
end

== matlab function sim_tcyb_2024_att_ctrl/cal Gamma_Fi_min_dzetai agent 3 ==
  data: Gamma_Fi_vec input; Gamma_Fi_min_dzetai_3 output; d_zetai_vec input
function Gamma_Fi_min_dzetai_3 = fcn(Gamma_Fi_vec, d_zetai_vec)
%%%% 计算矩阵 Gamma_Fi_min_dzetai
iiuav = 3;
Gamma_Fi_min_dzetai_3 = zeros(3,6);
Gamma_Fi_min_dzetai_3(1,1) = Gamma_Fi_vec(1,1) - d_zetai_vec(1,iiuav);
Gamma_Fi_min_dzetai_3(2,2) = Gamma_Fi_vec(2,2) - d_zetai_vec(2,iiuav);
Gamma_Fi_min_dzetai_3(3,3) = Gamma_Fi_vec(3,3) - d_zetai_vec(3,iiuav);
Gamma_Fi_min_dzetai_3(2,4) = Gamma_Fi_vec(2,4) - d_zetai_vec(3,iiuav);
Gamma_Fi_min_dzetai_3(3,4) = Gamma_Fi_vec(3,4) - d_zetai_vec(2,iiuav);
Gamma_Fi_min_dzetai_3(1,5) = Gamma_Fi_vec(1,5) - d_zetai_vec(3,iiuav);
Gamma_Fi_min_dzetai_3(3,5) = Gamma_Fi_vec(3,5) - d_zetai_vec(1,iiuav);
Gamma_Fi_min_dzetai_3(1,6) = Gamma_Fi_vec(1,6) - d_zetai_vec(2,iiuav);
Gamma_Fi_min_dzetai_3(2,6) = Gamma_Fi_vec(2,6) - d_zetai_vec(1,iiuav);
end

== matlab function sim_tcyb_2024_att_ctrl/cal Gamma_Fi_min_dzetai agent 4 ==
  data: Gamma_Fi_vec input; Gamma_Fi_min_dzetai_4 output; d_zetai_vec input
function Gamma_Fi_min_dzetai_4 = fcn(Gamma_Fi_vec, d_zetai_vec)
%%%% 计算矩阵 Gamma_Fi_min_dzetai
iiuav = 4;
Gamma_Fi_min_dzetai_4 = zeros(3,6);
Gamma_Fi_min_dzetai_4(1,1) = Gamma_Fi_vec(1,1) - d_zetai_vec(1,iiuav);
Gamma_Fi_min_dzetai_4(2,2) = Gamma_Fi_vec(2,2) - d_zetai_vec(2,iiuav);
Gamma_Fi_min_dzetai_4(3,3) = Gamma_Fi_vec(3,3) - d_zetai_vec(3,iiuav);
Gamma_Fi_min_dzetai_4(2,4) = Gamma_Fi_vec(2,4) - d_zetai_vec(3,iiuav);
Gamma_Fi_min_dzetai_4(3,4) = Gamma_Fi_vec(3,4) - d_zetai_vec(2,iiuav);
Gamma_Fi_min_dzetai_4(1,5) = Gamma_Fi_vec(1,5) - d_zetai_vec(3,iiuav);
Gamma_Fi_min_dzetai_4(3,5) = Gamma_Fi_vec(3,5) - d_zetai_vec(1,iiuav);
Gamma_Fi_min_dzetai_4(1,6) = Gamma_Fi_vec(1,6) - d_zetai_vec(2,iiuav);
Gamma_Fi_min_dzetai_4(2,6) = Gamma_Fi_vec(2,6) - d_zetai_vec(1,iiuav);
end

== matlab function sim_tcyb_2024_att_ctrl/cal Gamma_Fi_min_dzetai agent 5 ==
  data: Gamma_Fi_vec input; Gamma_Fi_min_dzetai_5 output; d_zetai_vec input
function Gamma_Fi_min_dzetai_5 = fcn(Gamma_Fi_vec, d_zetai_vec)
%%%% 计算矩阵 Gamma_Fi_min_dzetai
iiuav = 5;
Gamma_Fi_min_dzetai_5 = zeros(3,6);
Gamma_Fi_min_dzetai_5(1,1) = Gamma_Fi_vec(1,1) - d_zetai_vec(1,iiuav);
Gamma_Fi_min_dzetai_5(2,2) = Gamma_Fi_vec(2,2) - d_zetai_vec(2,iiuav);
Gamma_Fi_min_dzetai_5(3,3) = Gamma_Fi_vec(3,3) - d_zetai_vec(3,iiuav);
Gamma_Fi_min_dzetai_5(2,4) = Gamma_Fi_vec(2,4) - d_zetai_vec(3,iiuav);
Gamma_Fi_min_dzetai_5(3,4) = Gamma_Fi_vec(3,4) - d_zetai_vec(2,iiuav);
Gamma_Fi_min_dzetai_5(1,5) = Gamma_Fi_vec(1,5) - d_zetai_vec(3,iiuav);
Gamma_Fi_min_dzetai_5(3,5) = Gamma_Fi_vec(3,5) - d_zetai_vec(1,iiuav);
Gamma_Fi_min_dzetai_5(1,6) = Gamma_Fi_vec(1,6) - d_zetai_vec(2,iiuav);
Gamma_Fi_min_dzetai_5(2,6) = Gamma_Fi_vec(2,6) - d_zetai_vec(1,iiuav);
end

== matlab function sim_tcyb_2024_att_ctrl/combine Gamma_Fi_min_dzetai ==
  data: Gamma_Fi_min_dzetai_1 input; Gamma_Fi_min_dzetai_2 input; Gamma_Fi_min_dzetai_3 input; Gamma_Fi_min_dzetai_4 input; Gamma_Fi_min_dzetai_5 input; Gamma_Fi_min_dzetai_vec output
function Gamma_Fi_min_dzetai_vec  = fcn(Gamma_Fi_min_dzetai_1, Gamma_Fi_min_dzetai_2, Gamma_Fi_min_dzetai_3, Gamma_Fi_min_dzetai_4, Gamma_Fi_min_dzetai_5)
%%%% 合并计算矩阵 Gamma_Fi_min_dzetai
Gamma_Fi_min_dzetai_vec = zeros(3,6,5);
Gamma_Fi_min_dzetai_vec(:,:,1) = Gamma_Fi_min_dzetai_1;
Gamma_Fi_min_dzetai_vec(:,:,2) = Gamma_Fi_min_dzetai_2;
Gamma_Fi_min_dzetai_vec(:,:,3) = Gamma_Fi_min_dzetai_3;
Gamma_Fi_min_dzetai_vec(:,:,4) = Gamma_Fi_min_dzetai_4;
Gamma_Fi_min_dzetai_vec(:,:,5) = Gamma_Fi_min_dzetai_5;

== matlab function sim_tcyb_2024_att_ctrl/cal thetai_hat agent 1 ==
  data: mu input; d_thetai_hat_1 output; wi_vec input; wei_vec input; zetai_vec input; Gamma_Fi_min_dzetai_vec input; Gamma_wi_vec input
function d_thetai_hat_1 = fcn(mu, wi_vec, wei_vec, zetai_vec, Gamma_Fi_min_dzetai_vec, Gamma_wi_vec)
%%%% 计算自适应律 thetai_hat
iiuav = 1;
d_thetai_hat_1 = mu * ( ( Gamma_Fi_min_dzetai_vec(:,:,iiuav) - cal_askew_mat( wi_vec(:,iiuav) ) * Gamma_wi_vec(:,:,iiuav) )' ) ...
                                        * ( wei_vec(:,iiuav) - zetai_vec(:,iiuav) );
end

== matlab function sim_tcyb_2024_att_ctrl/cal Rei agent 1 ==
  data: Rei_1 output; sgei_vec input
function Rei_1 = fcn(sgei_vec)
%%%% 由罗德里格常量sgi求解姿态旋转矩阵Ri
iiuav = 1;
Rei_1 = eye(3) + 4 * ( 1 - ( ( ( sgei_vec(:,iiuav)' ) * sgei_vec(:,iiuav) ) / ( ( 1 + ( sgei_vec(:,iiuav)' ) * sgei_vec(:,iiuav) ) ^ 2 ) ) ) * cal_askew_mat( sgei_vec(:,iiuav) ) ...
                            + ( 8 / ( ( 1 + ( sgei_vec(:,iiuav)' ) * sgei_vec(:,iiuav) ) ^ 2 ) ) * cal_askew_mat( sgei_vec(:,iiuav) ) * cal_askew_mat( sgei_vec(:,iiuav) );
Rei_1 = Rei_1';
end

== matlab function sim_tcyb_2024_att_ctrl/cal thetai_hat agent 2 ==
  data: mu input; d_thetai_hat_2 output; wi_vec input; wei_vec input; zetai_vec input; Gamma_Fi_min_dzetai_vec input; Gamma_wi_vec input
function d_thetai_hat_2 = fcn(mu, wi_vec, wei_vec, zetai_vec, Gamma_Fi_min_dzetai_vec, Gamma_wi_vec)
%%%% 计算自适应律 thetai_hat
iiuav = 2;
d_thetai_hat_2 = mu * ( ( Gamma_Fi_min_dzetai_vec(:,:,iiuav) - cal_askew_mat( wi_vec(:,iiuav) ) * Gamma_wi_vec(:,:,iiuav) )' ) ...
                                        * ( wei_vec(:,iiuav) - zetai_vec(:,iiuav) );
end

== matlab function sim_tcyb_2024_att_ctrl/cal thetai_hat agent 3 ==
  data: mu input; d_thetai_hat_3 output; wi_vec input; wei_vec input; zetai_vec input; Gamma_Fi_min_dzetai_vec input; Gamma_wi_vec input
function d_thetai_hat_3 = fcn(mu, wi_vec, wei_vec, zetai_vec, Gamma_Fi_min_dzetai_vec, Gamma_wi_vec)
%%%% 计算自适应律 thetai_hat
iiuav = 3;
d_thetai_hat_3 = mu * ( ( Gamma_Fi_min_dzetai_vec(:,:,iiuav) - cal_askew_mat( wi_vec(:,iiuav) ) * Gamma_wi_vec(:,:,iiuav) )' ) ...
                                        * ( wei_vec(:,iiuav) - zetai_vec(:,iiuav) );
end

== matlab function sim_tcyb_2024_att_ctrl/cal thetai_hat agent 4 ==
  data: mu input; d_thetai_hat_4 output; wi_vec input; wei_vec input; zetai_vec input; Gamma_Fi_min_dzetai_vec input; Gamma_wi_vec input
function d_thetai_hat_4 = fcn(mu, wi_vec, wei_vec, zetai_vec, Gamma_Fi_min_dzetai_vec, Gamma_wi_vec)
%%%% 计算自适应律 thetai_hat
iiuav = 4;
d_thetai_hat_4 = mu * ( ( Gamma_Fi_min_dzetai_vec(:,:,iiuav) - cal_askew_mat( wi_vec(:,iiuav) ) * Gamma_wi_vec(:,:,iiuav) )' ) ...
                                        * ( wei_vec(:,iiuav) - zetai_vec(:,iiuav) );
end

== matlab function sim_tcyb_2024_att_ctrl/cal thetai_hat agent 5 ==
  data: mu input; d_thetai_hat_5 output; wi_vec input; wei_vec input; zetai_vec input; Gamma_Fi_min_dzetai_vec input; Gamma_wi_vec input
function d_thetai_hat_5 = fcn(mu, wi_vec, wei_vec, zetai_vec, Gamma_Fi_min_dzetai_vec, Gamma_wi_vec)
%%%% 计算自适应律 thetai_hat
iiuav = 5;
d_thetai_hat_5 = mu * ( ( Gamma_Fi_min_dzetai_vec(:,:,iiuav) - cal_askew_mat( wi_vec(:,iiuav) ) * Gamma_wi_vec(:,:,iiuav) )' ) ...
                                        * ( wei_vec(:,iiuav) - zetai_vec(:,iiuav) );
end

== matlab function sim_tcyb_2024_att_ctrl/combine thetai_hat ==
  data: thetai_hat_1 input; thetai_hat_2 input; thetai_hat_3 input; thetai_hat_4 input; thetai_hat_5 input; thetai_hat_vec output
function thetai_hat_vec  = fcn(thetai_hat_1, thetai_hat_2, thetai_hat_3, thetai_hat_4, thetai_hat_5)
%%%% 合并自适应律 thetai_hat
thetai_hat_vec = zeros(6,5);
thetai_hat_vec(:,1) = thetai_hat_1(:);
thetai_hat_vec(:,2) = thetai_hat_2(:);
thetai_hat_vec(:,3) = thetai_hat_3(:);
thetai_hat_vec(:,4) = thetai_hat_4(:);
thetai_hat_vec(:,5) = thetai_hat_5(:);

== matlab function sim_tcyb_2024_att_ctrl/cal taui agent 2 ==
  data: kw input; ksg input; tau_2 output; wi_vec input; wei_vec input; zetai_vec input; sgei_vec input; dw_hat_vec input; thetai_hat_vec input; Gamma_wi_vec input; Gamma_Fi_min_dzetai_vec input
function tau_2 = fcn(kw, ksg, wi_vec, wei_vec, zetai_vec, sgei_vec, dw_hat_vec, ...
                                        thetai_hat_vec, Gamma_wi_vec, Gamma_Fi_min_dzetai_vec)
%%%% 计算用于姿态控制的驱动力矩控制输入
iiuav = 2;
tau_2 = -kw * ( wei_vec(:,iiuav) - zetai_vec(:,iiuav) ) - ksg * sgei_vec(:,iiuav) - dw_hat_vec(:,iiuav) ...
                - ( Gamma_Fi_min_dzetai_vec(:,:,iiuav) - cal_askew_mat( wi_vec(:,iiuav) ) * Gamma_wi_vec(:,:,iiuav) ) * thetai_hat_vec(:,iiuav);
end

== matlab function sim_tcyb_2024_att_ctrl/E_sgei agent 2 ==
  data: sgei_vec input; E_sgei_2 output
function E_sgei_2 = fcn(sgei_vec)
%%%% 更新四元数微分方程
iiuav = 2;
E_sgei_2 = (1/4) * ( ( 1 - (sgei_vec(:,iiuav)') * sgei_vec(:,iiuav) ) * eye(3) ...
                    + 2 * cal_askew_mat( sgei_vec(:,iiuav) ) + 2 * sgei_vec(:,iiuav) * ( sgei_vec(:,iiuav)' ) );
end

== matlab function sim_tcyb_2024_att_ctrl/cal taui agent 3 ==
  data: kw input; ksg input; tau_3 output; wi_vec input; wei_vec input; zetai_vec input; sgei_vec input; dw_hat_vec input; thetai_hat_vec input; Gamma_wi_vec input; Gamma_Fi_min_dzetai_vec input
function tau_3 = fcn(kw, ksg, wi_vec, wei_vec, zetai_vec, sgei_vec, dw_hat_vec, ...
                                        thetai_hat_vec, Gamma_wi_vec, Gamma_Fi_min_dzetai_vec)
%%%% 计算用于姿态控制的驱动力矩控制输入
iiuav = 3;
tau_3 = -kw * ( wei_vec(:,iiuav) - zetai_vec(:,iiuav) ) - ksg * sgei_vec(:,iiuav) - dw_hat_vec(:,iiuav) ...
                - ( Gamma_Fi_min_dzetai_vec(:,:,iiuav) - cal_askew_mat( wi_vec(:,iiuav) ) * Gamma_wi_vec(:,:,iiuav) ) * thetai_hat_vec(:,iiuav);
end

== matlab function sim_tcyb_2024_att_ctrl/cal taui agent 4 ==
  data: kw input; ksg input; tau_4 output; wi_vec input; wei_vec input; zetai_vec input; sgei_vec input; dw_hat_vec input; thetai_hat_vec input; Gamma_wi_vec input; Gamma_Fi_min_dzetai_vec input
function tau_4 = fcn(kw, ksg, wi_vec, wei_vec, zetai_vec, sgei_vec, dw_hat_vec, ...
                                        thetai_hat_vec, Gamma_wi_vec, Gamma_Fi_min_dzetai_vec)
%%%% 计算用于姿态控制的驱动力矩控制输入
iiuav = 4;
tau_4 = -kw * ( wei_vec(:,iiuav) - zetai_vec(:,iiuav) ) - ksg * sgei_vec(:,iiuav) - dw_hat_vec(:,iiuav) ...
                - ( Gamma_Fi_min_dzetai_vec(:,:,iiuav) - cal_askew_mat( wi_vec(:,iiuav) ) * Gamma_wi_vec(:,:,iiuav) ) * thetai_hat_vec(:,iiuav);
end

== matlab function sim_tcyb_2024_att_ctrl/cal taui agent 5 ==
  data: kw input; ksg input; tau_5 output; wi_vec input; wei_vec input; zetai_vec input; sgei_vec input; dw_hat_vec input; thetai_hat_vec input; Gamma_wi_vec input; Gamma_Fi_min_dzetai_vec input
function tau_5 = fcn(kw, ksg, wi_vec, wei_vec, zetai_vec, sgei_vec, dw_hat_vec, ...
                                        thetai_hat_vec, Gamma_wi_vec, Gamma_Fi_min_dzetai_vec)
%%%% 计算用于姿态控制的驱动力矩控制输入
iiuav = 5;
tau_5 = -kw * ( wei_vec(:,iiuav) - zetai_vec(:,iiuav) ) - ksg * sgei_vec(:,iiuav) - dw_hat_vec(:,iiuav) ...
                - ( Gamma_Fi_min_dzetai_vec(:,:,iiuav) - cal_askew_mat( wi_vec(:,iiuav) ) * Gamma_wi_vec(:,:,iiuav) ) * thetai_hat_vec(:,iiuav);
end

== matlab function sim_tcyb_2024_att_ctrl/cal Rci agent 1 ==
  data: Ri_vec input; Rci_1 output; Rei_vec input
function Rci_1 = fcn(Ri_vec, Rei_vec)
%%%% 更新姿态旋转指令矩阵
iiuav = 1;
Rci_1 = Ri_vec(:,:,iiuav) * ( Rei_vec(:,:,iiuav)' );
end

== matlab function sim_tcyb_2024_att_ctrl/cal Rei agent 2 ==
  data: Rei_2 output; sgei_vec input
function Rei_2 = fcn(sgei_vec)
%%%% 由罗德里格常量sgi求解姿态旋转矩阵Ri
iiuav = 2;
Rei_2 = eye(3) + 4 * ( 1 - ( ( ( sgei_vec(:,iiuav)' ) * sgei_vec(:,iiuav) ) / ( ( 1 + ( sgei_vec(:,iiuav)' ) * sgei_vec(:,iiuav) ) ^ 2 ) ) ) * cal_askew_mat( sgei_vec(:,iiuav) ) ...
                            + ( 8 / ( ( 1 + ( sgei_vec(:,iiuav)' ) * sgei_vec(:,iiuav) ) ^ 2 ) ) * cal_askew_mat( sgei_vec(:,iiuav) ) * cal_askew_mat( sgei_vec(:,iiuav) );
Rei_2 = Rei_2';
end

== matlab function sim_tcyb_2024_att_ctrl/cal Rci agent 2 ==
  data: Ri_vec input; Rci_2 output; Rei_vec input
function Rci_2 = fcn(Ri_vec, Rei_vec)
%%%% 更新姿态旋转指令矩阵
iiuav = 2;
Rci_2 = Ri_vec(:,:,iiuav) * ( Rei_vec(:,:,iiuav)' );
end

== matlab function sim_tcyb_2024_att_ctrl/cal Rci agent 3 ==
  data: Ri_vec input; Rci_3 output; Rei_vec input
function Rci_3 = fcn(Ri_vec, Rei_vec)
%%%% 更新姿态旋转指令矩阵
iiuav = 3;
Rci_3 = Ri_vec(:,:,iiuav) * ( Rei_vec(:,:,iiuav)' );
end

== matlab function sim_tcyb_2024_att_ctrl/cal Rci agent 4 ==
  data: Ri_vec input; Rci_4 output; Rei_vec input
function Rci_4 = fcn(Ri_vec, Rei_vec)
%%%% 更新姿态旋转指令矩阵
iiuav = 4;
Rci_4 = Ri_vec(:,:,iiuav) * ( Rei_vec(:,:,iiuav)' );
end

== matlab function sim_tcyb_2024_att_ctrl/cal Rci agent 5 ==
  data: Ri_vec input; Rci_5 output; Rei_vec input
function Rci_5 = fcn(Ri_vec, Rei_vec)
%%%% 更新姿态旋转指令矩阵
iiuav = 5;
Rci_5 = Ri_vec(:,:,iiuav) * ( Rei_vec(:,:,iiuav)' );
end

== matlab function sim_tcyb_2024_att_ctrl/combine Rci ==
  data: Rci_1 input; Rci_vec output; Rci_2 input; Rci_3 input; Rci_4 input; Rci_5 input
function Rci_vec = fcn(Rci_1, Rci_2, Rci_3, Rci_4, Rci_5)
%%%% 合并姿态计算矩阵
Rci_vec = zeros(3,3,5);
Rci_vec(:,:,1) = Rci_1;
Rci_vec(:,:,2) = Rci_2;
Rci_vec(:,:,3) = Rci_3;
Rci_vec(:,:,4) = Rci_4;
Rci_vec(:,:,5) = Rci_5;

== matlab function sim_tcyb_2024_att_ctrl/depart zetai_5 ==
  data: y output; x input
function y = fcn(x)
y = x(:,5);

end

== matlab function sim_tcyb_2024_att_ctrl/depart zetai_1 ==
  data: y output; x input
function y = fcn(x)
y = x(:,1);

end

== matlab function sim_tcyb_2024_att_ctrl/depart zetai_2 ==
  data: y output; x input
function y = fcn(x)
y = x(:,2);

end

== matlab function sim_tcyb_2024_att_ctrl/depart zetai_3 ==
  data: y output; x input
function y = fcn(x)
y = x(:,3);

end

== matlab function sim_tcyb_2024_att_ctrl/cal wei agent 2 ==
  data: wi_vec input; wei_2 output; Rei_vec input; wci_vec input
function wei_2 = fcn(wi_vec, Rei_vec, wci_vec)
%%%% 更新姿态角速率误差
iiuav = 2;
wei_2 = wi_vec(:,iiuav) - (Rei_vec(:,:,iiuav)') * wci_vec(:,iiuav);
end

== matlab function sim_tcyb_2024_att_ctrl/depart zetai_4 ==
  data: y output; x input
function y = fcn(x)
y = x(:,4);

end

== matlab function sim_tcyb_2024_att_ctrl/depart theta_hat_5 ==
  data: y output; x input
function y = fcn(x)
y = x(:,5);

end

== matlab function sim_tcyb_2024_att_ctrl/depart theta_hat_1 ==
  data: y output; x input
function y = fcn(x)
y = x(:,1);

end

== matlab function sim_tcyb_2024_att_ctrl/cal combine sigma_bar_w_tilt ==
  data: sigma_bar_w_vec input; sigma_bar_w_hat_vec input; sigma_bar_w_tilt_vec output
function sigma_bar_w_tilt_vec = fcn(sigma_bar_w_vec, sigma_bar_w_hat_vec)
%%%% 计算虚拟速度观测误差sigma_bar_w_tilt
sigma_bar_w_tilt_vec = zeros(3,5);
for iiuav = 1:5
    sigma_bar_w_tilt_vec(:,iiuav) = sigma_bar_w_vec(:,iiuav) - sigma_bar_w_hat_vec(:,iiuav);
end

== matlab function sim_tcyb_2024_att_ctrl/cal differentiator d_sigma_bar_w_hat agent 3/cal sig3 ==
  data: x input; z output; y input
function z = fcn(x, y)
z = x(:) .* sign(y(:));

== matlab function sim_tcyb_2024_att_ctrl/cal differentiator d_sigma_bar_w_hat agent 3/cal sig4 ==
  data: x input; z output; y input
function z = fcn(x, y)
z = x(:) .* sign(y(:));

== matlab function sim_tcyb_2024_att_ctrl/cal wei agent 1 ==
  data: wi_vec input; wei_1 output; Rei_vec input; wci_vec input
function wei_1 = fcn(wi_vec, Rei_vec, wci_vec)
%%%% 更新姿态角速率误差
iiuav = 1;
wei_1 = wi_vec(:,iiuav) - (Rei_vec(:,:,iiuav)') * wci_vec(:,iiuav);
end

== matlab function sim_tcyb_2024_att_ctrl/dsgei dynam agent 1 ==
  data: E_sgei_vec input; dsgei_1 output; wei_vec input
function dsgei_1 = fcn(E_sgei_vec, wei_vec)
%%%% 更新四元数误差微分方程
iiuav = 1;
dsgei_1 = E_sgei_vec(:,:,iiuav) * wei_vec(:,iiuav);
end

== matlab function sim_tcyb_2024_att_ctrl/depart theta_hat_2 ==
  data: y output; x input
function y = fcn(x)
y = x(:,2);

end

== matlab function sim_tcyb_2024_att_ctrl/depart theta_hat_3 ==
  data: y output; x input
function y = fcn(x)
y = x(:,3);

end

== matlab function sim_tcyb_2024_att_ctrl/cal differentiator d_sigma_bar_w_hat agent 3/cal sig5 ==
  data: x input; z output; y input
function z = fcn(x, y)
z = x(:) .* sign(y(:));

== matlab function sim_tcyb_2024_att_ctrl/depart theta_hat_4 ==
  data: y output; x input
function y = fcn(x)
y = x(:,4);

end

== matlab function sim_tcyb_2024_att_ctrl/cal Ri agent 3 ==
  data: Ri_3 output; sgi_vec input
function Ri_3 = fcn(sgi_vec)
%%%% 由罗德里格常量sgi求解姿态旋转矩阵Ri
iiuav = 3;
Ri_3 = eye(3) + 4 * ( 1 - ( ( ( sgi_vec(:,iiuav)' ) * sgi_vec(:,iiuav) ) / ( ( 1 + ( sgi_vec(:,iiuav)' ) * sgi_vec(:,iiuav) ) ^ 2 ) ) ) * cal_askew_mat( sgi_vec(:,iiuav) ) ...
                            + ( 8 / ( ( 1 + ( sgi_vec(:,iiuav)' ) * sgi_vec(:,iiuav) ) ^ 2 ) ) * cal_askew_mat( sgi_vec(:,iiuav) ) * cal_askew_mat( sgi_vec(:,iiuav) );
Ri_3 = Ri_3';
end

== matlab function sim_tcyb_2024_att_ctrl/depart Ji_1_1 ==
  data: y output; x input
function y = fcn(x)
y = x(1,1);
end

== matlab function sim_tcyb_2024_att_ctrl/depart Ji_2_2 ==
  data: y output; x input
function y = fcn(x)
y = x(2,2);
end

== matlab function sim_tcyb_2024_att_ctrl/depart Ji_3_3 ==
  data: y output; x input
function y = fcn(x)
y = x(3,3);
end

== matlab function sim_tcyb_2024_att_ctrl/depart Ji_2_3 ==
  data: y output; x input
function y = fcn(x)
y = x(2,3);
end

== matlab function sim_tcyb_2024_att_ctrl/depart Ji_1_3 ==
  data: y output; x input
function y = fcn(x)
y = x(1,3);
end

== matlab function sim_tcyb_2024_att_ctrl/depart Ji_1_2 ==
  data: y output; x input
function y = fcn(x)
y = x(1,2);
end
